simulink model "InjectorShellModel"  (R2019a)
settings: Solver=VariableStepAuto  StartTime=0.0  StopTime=10.0  RelTol=1e-3
settings Model: Creator=Dipak  LastModifiedBy=Dipak

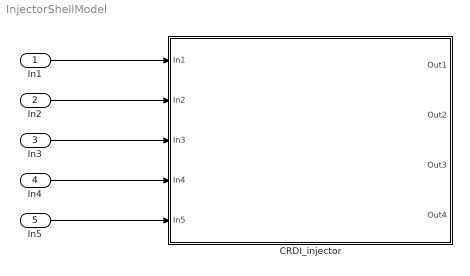
== system InjectorShellModel ==
  In1 : Inport
  In2 : Inport  Port=2
  In3 : Inport  Port=3
  In4 : Inport  Port=4
  In5 : Inport  Port=5
  CRDI_injector : Subsystem
  wires:
  In1/1 -> CRDI_injector/1(In1)
  In2/1 -> CRDI_injector/2(In2)
  In3/1 -> CRDI_injector/3(In3)
  In4/1 -> CRDI_injector/4(In4)
  In5/1 -> CRDI_injector/5(In5)

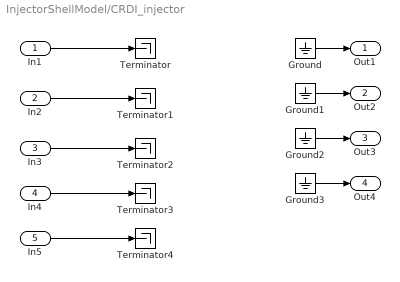
== system InjectorShellModel/CRDI_injector ==
  In1 : Inport
  In2 : Inport  Port=2
  In3 : Inport  Port=3
  In4 : Inport  Port=4
  In5 : Inport  Port=5
  Ground{,1..3} (4 alike) : Ground
  Terminator{,1..4} (5 alike) : Terminator
  Out1 : Outport
  Out2 : Outport  Port=2
  Out3 : Outport  Port=3
  Out4 : Outport  Port=4
  wires:
  Ground/1 -> Out1/1
  In1/1 -> Terminator/1
  In2/1 -> Terminator1/1
  In3/1 -> Terminator2/1
  Ground1/1 -> Out2/1
  Ground2/1 -> Out3/1
  Ground3/1 -> Out4/1
  In4/1 -> Terminator3/1
  In5/1 -> Terminator4/1
